simulink model "ControlAdapter"  (R2023a)
settings: Solver=VariableStepAuto  StartTime=0.0  StopTime=10.0  RelTol=1e-3
settings Model: Creator=Waffle  LastModifiedBy=Waffle

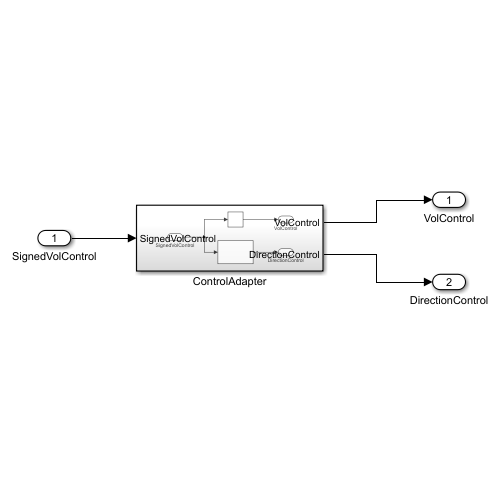
[thumbnail: Simulink's stored preview of the top-level diagram]
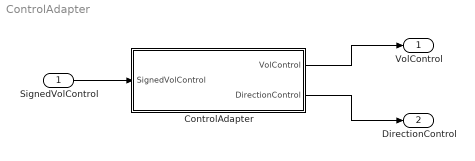
== system ControlAdapter ==
  SignedVolControl : Inport
  ControlAdapter : Subsystem
  VolControl : Outport
  DirectionControl : Outport  Port=2  OutDataTypeStr=boolean
  wires:
  SignedVolControl/1 -> ControlAdapter/1(SignedVolControl)
  ControlAdapter/1(VolControl) -> VolControl/1
  ControlAdapter/2(DirectionControl) -> DirectionControl/1

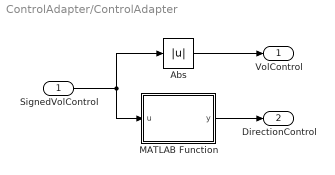
== system ControlAdapter/ControlAdapter ==
  SignedVolControl : Inport
  Abs : Abs  SaturateOnIntegerOverflow=off
  MATLAB Function : MATLAB Function  TreatAsAtomicUnit=on
  VolControl : Outport
  DirectionControl : Outport  Port=2  OutDataTypeStr=boolean
  wires:
  Abs/1 -> VolControl/1
  SignedVolControl/1 -> MATLAB Function/1(u), Abs/1
  MATLAB Function/1(y) -> DirectionControl/1

== matlab function ControlAdapter/MATLAB Function ==
  data: u input; y output
function y = fcn(u)
if u>0
    y=true;
else
    y=false;
end
